simulink model "barker7_correlator"  (R2012b)
settings: Solver=ode45  StartTime=0.0  StopTime=5  RelTol=1e-3
settings Model: Creator=jeldon  LastModifiedBy=JohnE
settings DataIOCC: SignalLoggingSaveFormat=ModelDataLogs  SignalLogging=off
settings OptimizationCC: BlockReduction=off  ConditionallyExecuteInputs=off  InlineParams=on
settings DebuggingCC: AlgebraicLoopMsg=error  FcnCallInpInsideContextMsg=EnableAllAsWarning
settings HardwareCC: ProdHWDeviceType=ASIC/FPGA->ASIC/FPGA  ProdEqTarget=off

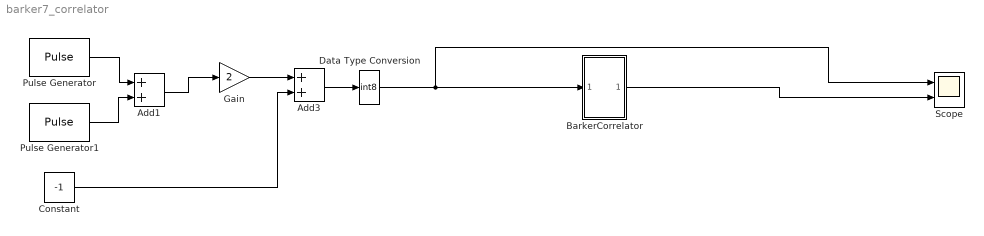
== system barker7_correlator ==
  Add1 : Sum
  Add3 : Sum
  BarkerCorrelator : Subsystem
  Constant : Constant  Value=-1
  Data Type Conversion : DataTypeConversion  OutDataTypeStr=int8
  Gain : Gain  Gain=2  OutDataTypeStr=Inherit: Same as input
  Pulse Generator : DiscretePulseGenerator  Period=100  PhaseDelay=9  SampleTime=0.01
  Pulse Generator1 : DiscretePulseGenerator  Period=100  PulseWidth=3  PhaseDelay=4  SampleTime=0.01
  Scope : Scope  NumInputPorts=2
      settings: YMin=-5~-5  YMax=5~7.1
  wires:
  Pulse Generator/1 -> Add1/1
  Pulse Generator1/1 -> Add1/2
  Data Type Conversion/1 -> BarkerCorrelator/1(In1), Scope/1
  Add1/1 -> Gain/1
  Gain/1 -> Add3/1
  Add3/1 -> Data Type Conversion/1
  Constant/1 -> Add3/2
  BarkerCorrelator/1(Out1) -> Scope/2

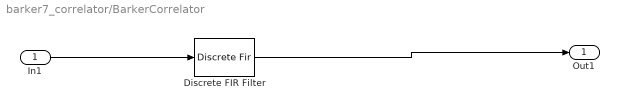
== system barker7_correlator/BarkerCorrelator ==
  In1 : Inport
  Discrete FIR Filter : DiscreteFir  FilterStructure=Direct form transposed  Coefficients=[-1 1 -1 -1 1 1 1 ]  AccumDataTypeStr=int8  OutDataTypeStr=int8
  Out1 : Outport
  wires:
  Discrete FIR Filter/1 -> Out1/1
  In1/1 -> Discrete FIR Filter/1
